simulink model "boost_simulink_copy"  (R2021a)
settings: Solver=FixedStepDiscrete  StartTime=0.0  StopTime=0.5  FixedStep=sampleTime  MaxStep=1e-4  RelTol=1e-4  EnableMultiTasking=on
InitFcn:
  | boost_parameters
model workspace (MAT data in the model file):
  Phase1 = 0
values from neighbouring files (symbols this model uses):
  CoutModulesp = 271e-6    (= 0.000271)    [boost_parameters.m]    (also in unbalance_boost.m)
  D = (1-Vin/Vout)    (= 0.25)    [boost_parameters.m]    (also in calculations.m = (1-VinOneModule/VoutOneModule); flying_capacitor_parameters.m; unbalance_boost.m)
  Lcoilsp = 0.517e-3    (= 0.000517)    [boost_parameters.m]    (also in unbalance_boost.m = 0.001034)
  ModuleAPhase = 0    [boost_parameters.m]    (also in flying_capacitor_parameters.m = 90; unbalance_boost.m)
  ModuleBPhase = 180    [boost_parameters.m]    (also in flying_capacitor_parameters.m = 270; unbalance_boost.m = 90)
  ModuleCPhase = 180    [boost_parameters.m]    (also in flying_capacitor_parameters.m = 0)
  ModuleDPhase = 180    [boost_parameters.m]    (also in flying_capacitor_parameters.m)
  Rcoil = 1e-3    (= 0.001)    [boost_parameters.m]    (also in unbalance_boost.m)
  sampleTime = 5e-8    (= 5e-08)    [boost_parameters.m]    (also in flying_capacitor_parameters.m = 5e-07; unbalance_boost.m)
  Vin = 900    [boost_parameters.m]    (also in flying_capacitor_parameters.m; main.m = 880; unbalance_boost.m)
libraries: spsSeriesRLCBranchLib x35, spsVoltageMeasurementLib x32, spsCurrentMeasurementLib x27, spsDiodeLib x14, spsIGBTDiodeLib x14, simulink x10, spsDCVoltageSourceLib x7, spsTriangleGeneratorLib x5, spspowerguiLib x2
settings Model: Creator=The MathWorks, Inc.  LastModifiedBy=enes_
settings SolverCC: AlgebraicLoopSolver=TrustRegion  SolverResetMethod=Robust
settings OptimizationCC: EfficientFloat2IntCast=on  LifeSpan=inf
settings DebuggingCC: ReadBeforeWriteMsg=DisableAll  WriteAfterWriteMsg=DisableAll  WriteAfterReadMsg=DisableAll  UniqueDataStoreMsg=error  StrictBusMsg=ErrorOnBusTreatedAsVector  SFUnexpectedBacktrackingDiag=warning  SFNoUnconditionalDefaultTransitionDiag=warning  SFExecutionAtInitializationDiag=none  SFMachineParentedDataDiag=warning  ArithmeticOperatorsInVariantConditions=warning
settings ModelReferenceCC: UpdateModelReferenceTargets=IfOutOfDate
settings SFSimCC: SFSimEcho=off  SimUseLocalCustomCode=off  CustomCodeUndefinedFunction=UseInterfaceOnly
settings RTWCC: RTWUseLocalCustomCode=off
settings CodeAppCC: StateflowObjectComments=on
settings GRTTargetCC: TargetLangStandard=C89/C90 (ANSI)
settings ConfigComp: CovMetricSettings=dw  CovSaveCumulativeToWorkspaceVar=on  CovSaveSingleToWorkspaceVar=on  CovExternalEMLEnable=off
settings SimscapeCC: SimscapeNormalizeSystem=off  SimscapeNominalValues={1, 'bar'; 1, 'cm^3/s'; 1, 'bar*kg/s'; 1, 'kJ/kg'; 1, 'kW'; }

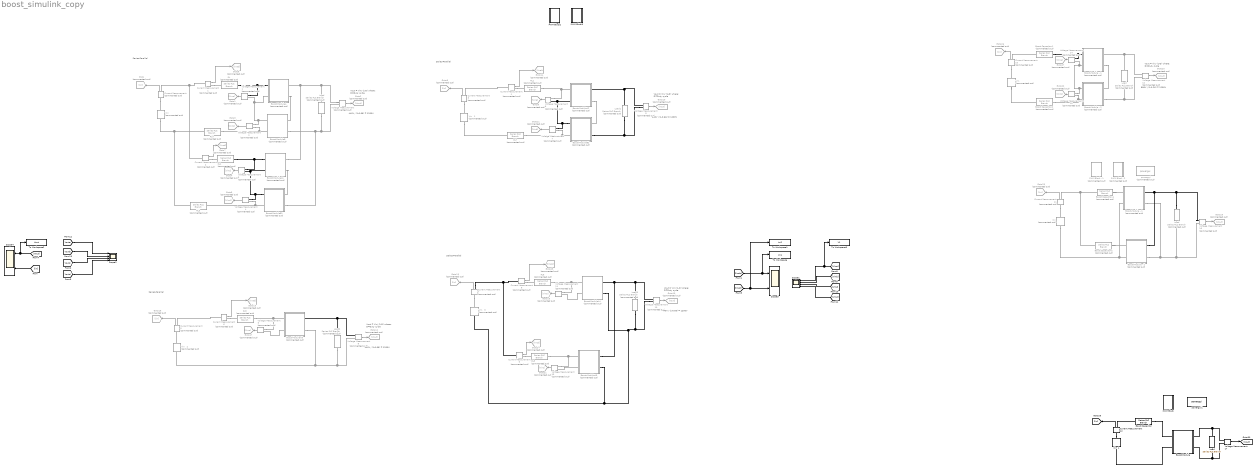
== system boost_simulink_copy ==
  note: Series-Parallel
  note: Vout = Vin/ (1-D)
      | where: D=Duty cycle
  note: 440V / (1-0.66) = 1200V
  note: Series-Parallel
  note: Vout = Vin/ (1-D)
      | where: D=Duty cycle
  note: 440V / (1-0.66) = 1200V
  note: 440V / (1-0.66) = 1200V
  note: Vout = Vin/ (1-D)
      | where: D=Duty cycle
  note: Series-Parallel
  note: Series-Parallel
  note: Vout = Vin/ (1-D)
      | where: D=Duty cycle
  note: 440V / (1-0.66) = 1200V
  note: 880V / (1-0.26) = 1200V
  note: Vout = Vin/ (1-D)
      | where: D=Duty cycle
  "Boost Capacitor   " : spsSeriesRLCBranchLib/Series RLC Branch  LConnTagsString=__new0  RConnTagsString=__new0  BranchType=L  Resistance=Rcoil  Inductance=Lcoilsp*2  SetiL0=off  InitialCurrent=8  Capacitance=1e-6  Setx0=off  InitialVoltage=0  Measurements=None
  Boost Capacitor-1 : spsSeriesRLCBranchLib/Series RLC Branch  Commented=on  LConnTagsString=__new0  RConnTagsString=__new0  BranchType=L  Resistance=Rcoil  Inductance=Lcoilsp/2  SetiL0=off  InitialCurrent=8  Capacitance=1e-6  Setx0=off  InitialVoltage=0  Measurements=None
  "Boost Capacitor-1  " : spsSeriesRLCBranchLib/Series RLC Branch  Commented=on  LConnTagsString=__new0  RConnTagsString=__new0  BranchType=L  Resistance=Rcoil  Inductance=Lcoilsp*2  SetiL0=off  InitialCurrent=8  Capacitance=1e-6  Setx0=off  InitialVoltage=0  Measurements=None
  Boost Capacitor-2 : spsSeriesRLCBranchLib/Series RLC Branch  Commented=on  LConnTagsString=__new0  RConnTagsString=__new0  BranchType=L  Resistance=Rcoil  Inductance=Lcoilsp/2  SetiL0=off  InitialCurrent=8  Capacitance=1e-6  Setx0=off  InitialVoltage=0  Measurements=None
  "Boost Capacitor-2   " : spsSeriesRLCBranchLib/Series RLC Branch  Commented=on  LConnTagsString=__new0  RConnTagsString=__new0  BranchType=L  Resistance=Rcoil  Inductance=Lcoilsp*2  SetiL0=off  InitialCurrent=8  Capacitance=1e-6  Setx0=off  InitialVoltage=0  Measurements=None
  "Boost-Module      " : Subsystem
  Boost-Module - 1 : Subsystem  Commented=on
  "Boost-Module - 1  " : Subsystem  Commented=on
  Boost-Module - 2 : Subsystem  Commented=on
  "Boost-Module - 2  " : Subsystem  Commented=on
  Boost-ModuleA : Subsystem  Commented=on
  Boost-ModuleA1 : Subsystem  Commented=on
  Boost-ModuleA2 : Subsystem  Commented=on
  Boost-ModuleA3 : Subsystem  Commented=on
  Boost-ModuleA4 : Subsystem  Commented=on
  Boost-ModuleA5 : Subsystem  Commented=on
  Boost-ModuleB : Subsystem  Commented=on
  Boost-ModuleB1 : Subsystem  Commented=on
  Boost-ModuleB2 : Subsystem  Commented=on
  Current Measurement{,1..11} (12 alike) : spsCurrentMeasurementLib/Current Measurement  Commented=on  PhasorSimulation=off  OutputType=Complex  PSBequivalent=0
  Current Measurement12 : spsCurrentMeasurementLib/Current Measurement  PhasorSimulation=off  OutputType=Complex  PSBequivalent=0
  Goto{,8,13,16,25..26} (6 alike) : Goto  Commented=on  GotoTag=Iin
  Goto{1,9,17..18,27} (5 alike) : Goto  Commented=on  GotoTag=Vina
  Goto{2,10,12,19..20,29} (6 alike) : Goto  Commented=on  GotoTag=Vout
  Goto11 : Goto  Commented=on  GotoTag=Vinb
  Goto{6,14..15,23} (4 alike) : Goto  Commented=on  GotoTag=Iinab
  Goto21 : Goto  Commented=on  GotoTag=Vinc
  Goto22 : Goto  Commented=on  GotoTag=Vinb
  Goto24 : Goto  Commented=on  GotoTag=Iincd
  Goto3 : Goto  Commented=on  GotoTag=Vinb
  Goto4 : Goto  Commented=on  GotoTag=Vinc
  Goto5 : Goto  Commented=on  GotoTag=Vind
  Goto7 : Goto  Commented=on  GotoTag=Iincd
  Load{,1..3} (4 alike) : spsSeriesRLCBranchLib/Series RLC Branch  Commented=on  LConnTagsString=__new0  RConnTagsString=__new0  BranchType=R  Resistance=72  Inductance=200e-6  SetiL0=off  InitialCurrent=0  Capacitance=400e-6  Setx0=off  InitialVoltage=0  Measurements=None
  "Load  " : spsSeriesRLCBranchLib/Series RLC Branch  Commented=on  LConnTagsString=__new0  RConnTagsString=__new0  BranchType=R  Resistance=72  Inductance=200e-6  SetiL0=off  InitialCurrent=0  Capacitance=400e-6  Setx0=off  InitialVoltage=0  Measurements=None
  "Load    " : spsSeriesRLCBranchLib/Series RLC Branch  Commented=on  LConnTagsString=__new0  RConnTagsString=__new0  BranchType=R  Resistance=72  Inductance=200e-6  SetiL0=off  InitialCurrent=0  Capacitance=400e-6  Setx0=off  InitialVoltage=0  Measurements=None
  "Load     " : spsSeriesRLCBranchLib/Series RLC Branch  LConnTagsString=__new0  RConnTagsString=__new0  BranchType=R  Resistance=72  Inductance=200e-6  SetiL0=off  InitialCurrent=0  Capacitance=400e-6  Setx0=off  InitialVoltage=0  Measurements=None
  "PWM Block " : Subsystem
  PWM Block - 1 : Subsystem  Commented=on
  PWM Block - 2 : Subsystem  Commented=on
  PWM Block2 : Subsystem
  PWM Block3 : Subsystem
  RL{,1,3..4} (4 alike) : spsSeriesRLCBranchLib/Series RLC Branch  Commented=on  LConnTagsString=__new0  RConnTagsString=__new0  BranchType=L  Resistance=Rcoil  Inductance=Lcoilsp  SetiL0=off  InitialCurrent=8  Capacitance=1e-6  Setx0=off  InitialVoltage=0  Measurements=None
  RL2 : spsSeriesRLCBranchLib/Series RLC Branch  Commented=on  LConnTagsString=__new0  RConnTagsString=__new0  BranchType=L  Resistance=Rcoil  Inductance=Lcoilsp/2  SetiL0=off  InitialCurrent=8  Capacitance=1e-6  Setx0=off  InitialVoltage=0  Measurements=None
  RL5 : spsSeriesRLCBranchLib/Series RLC Branch  Commented=on  LConnTagsString=__new0  RConnTagsString=__new0  BranchType=L  Resistance=Rcoil  Inductance=Lcoilsp*2  SetiL0=off  InitialCurrent=8  Capacitance=1e-6  Setx0=off  InitialVoltage=0  Measurements=None
  RL6 : spsSeriesRLCBranchLib/Series RLC Branch  Commented=on  LConnTagsString=__new0  RConnTagsString=__new0  BranchType=L  Resistance=Rcoil  Inductance=Lcoilsp*2  SetiL0=off  InitialCurrent=8  Capacitance=1e-6  Setx0=off  InitialVoltage=0  Measurements=None
  RL7 : spsSeriesRLCBranchLib/Series RLC Branch  Commented=on  LConnTagsString=__new0  RConnTagsString=__new0  BranchType=L  Resistance=Rcoil  Inductance=Lcoilsp/2  SetiL0=off  InitialCurrent=8  Capacitance=1e-6  Setx0=off  InitialVoltage=0  Measurements=None
  RL8 : spsSeriesRLCBranchLib/Series RLC Branch  Commented=on  LConnTagsString=__new0  RConnTagsString=__new0  BranchType=L  Resistance=Rcoil  Inductance=Lcoilsp*2  SetiL0=off  InitialCurrent=8  Capacitance=1e-6  Setx0=off  InitialVoltage=0  Measurements=None
  Scope1 : Scope  NumInputPorts=4
  Scope2 : Scope  NumInputPorts=4
  Scope3 : Scope  NumInputPorts=2
  Scope4 : Scope  NumInputPorts=2
  To Workspace : ToWorkspace  VariableName=Im1  SaveFormat=Timeseries  SampleTime=-1
  To Workspace1 : ToWorkspace  VariableName=Im2  SaveFormat=Timeseries  SampleTime=-1
  To Workspace2 : ToWorkspace  VariableName=Vout  SaveFormat=Timeseries  SampleTime=-1
  To Workspace3 : ToWorkspace  VariableName=V1  SaveFormat=Timeseries  SampleTime=-1
  "Vin  " : spsDCVoltageSourceLib/DC Voltage Source  Commented=on  Amplitude=Vin  Measurements=None
  Vin   {,1..3} (4 alike) : spsDCVoltageSourceLib/DC Voltage Source  Commented=on  Amplitude=Vin  Measurements=None
  "Vin     " : spsDCVoltageSourceLib/DC Voltage Source  Commented=on  Amplitude=Vin  Measurements=None
  Vin  1 : spsDCVoltageSourceLib/DC Voltage Source  Amplitude=Vin  Measurements=None
  Voltage Measurement{,1..16} (17 alike) : spsVoltageMeasurementLib/Voltage Measurement  Commented=on  PhasorSimulation=off  OutputType=Complex  PSBequivalent=0
  Voltage Measurement17 : spsVoltageMeasurementLib/Voltage Measurement  PhasorSimulation=off  OutputType=Complex  PSBequivalent=0
  powergui : spspowerguiLib/powergui  Priority=1  Commented=on  SimulationMode=Discrete  SampleTime=sampleTime  frequency=60  Iterations=50  frequencyindice=0  Pbase=100e6  ErrMax=1e-4  UnitsV=kV  UnitsW=MW  buscounter=0  FunctionMessages=off  echomessages=off  EnableUseOfTLC=off  CurrentSourceSwitches=off  DisableSnubberDevices=off  DisableRonSwitches=off  DisableVfSwitches=off  DisplayEquations=off  AutomaticDiscreteSolvers=off  SolverType=Tustin/Backward Euler (TBE)  Interpol=off  ExternalGateDelay=off  methode=off  Ts=100  x0status=blocks  SPID=on  SwTol=0  HookPort=off  NonlinearTolerance=1e-4  nMaxIteration=100  ContinueOnMaxIteration=off  RestoreLinks=warning  ResistiveCurrentMeasurement=off  Frange=[0:2:500]  Ylog=off  Xlog=on  ShowGrid=off  save=off  variable=ZData  structure=0  ZoomFFT=off  StartTime=0.0  cycles=1  DisplayStyle=1  fundamental=60  FreqAxis=off  MaxFrequency=1000  frequencyindicesteady=1  RmsSteady=1  display=off
  powergui1 : spspowerguiLib/powergui  Priority=1  SimulationMode=Discrete  SampleTime=sampleTime  frequency=60  Iterations=50  frequencyindice=0  Pbase=100e6  ErrMax=1e-4  UnitsV=kV  UnitsW=MW  buscounter=0  FunctionMessages=off  echomessages=off  EnableUseOfTLC=off  CurrentSourceSwitches=off  DisableSnubberDevices=off  DisableRonSwitches=off  DisableVfSwitches=off  DisplayEquations=off  AutomaticDiscreteSolvers=off  SolverType=Tustin/Backward Euler (TBE)  Interpol=off  ExternalGateDelay=off  methode=off  Ts=100  x0status=blocks  SPID=on  SwTol=0  HookPort=off  NonlinearTolerance=1e-4  nMaxIteration=100  ContinueOnMaxIteration=off  RestoreLinks=warning  ResistiveCurrentMeasurement=off  Frange=[0:2:500]  Ylog=off  Xlog=on  ShowGrid=off  save=off  variable=ZData  structure=0  ZoomFFT=off  StartTime=0.0  cycles=1  DisplayStyle=1  fundamental=60  FreqAxis=off  MaxFrequency=1000  frequencyindicesteady=1  RmsSteady=1  display=off
  wires:
  [Vout] -> To Workspace2/1, Scope4/1  "Vout"
  [Iin] -> Scope4/2
  [Vina] -> To Workspace3/1, Scope1/1
  [Vinb] -> Scope1/2
  [Vinc] -> Scope1/3
  [Vind] -> Scope1/4
  [Iincd] -> To Workspace1/1, Scope3/2
  [Iinab] -> Scope3/1, To Workspace/1
  [Vouta] -> Scope2/1  "A"
  [Voutb] -> Scope2/2  "B"
  [Voutc] -> Scope2/3  "C"
  [Voutd] -> Scope2/4  "D"
  Current Measurement2/1 -> Goto7/1
  Current Measurement1/1 -> Goto6/1
  Voltage Measurement2/1 -> Goto3/1
  Voltage Measurement4/1 -> Goto5/1
  Voltage Measurement3/1 -> Goto4/1
  Voltage Measurement1/1 -> Goto1/1
  Current Measurement/1 -> Goto/1
  Voltage Measurement/1 -> Goto2/1
  Voltage Measurement7/1 -> Goto11/1
  Voltage Measurement5/1 -> Goto10/1
  Voltage Measurement6/1 -> Goto9/1
  Current Measurement3/1 -> Goto8/1
  Current Measurement4/1 -> Goto14/1
  Voltage Measurement8/1 -> Goto12/1
  Current Measurement6/1 -> Goto15/1
  Current Measurement5/1 -> Goto16/1
  Voltage Measurement9/1 -> Goto17/1
  Current Measurement9/1 -> Goto24/1
  Voltage Measurement10/1 -> Goto19/1
  Voltage Measurement11/1 -> Goto18/1
  Current Measurement7/1 -> Goto13/1
  Current Measurement8/1 -> Goto23/1
  Voltage Measurement13/1 -> Goto21/1
  Voltage Measurement15/1 -> Goto22/1
  Voltage Measurement14/1 -> Goto27/1
  Current Measurement10/1 -> Goto26/1
  Voltage Measurement12/1 -> Goto20/1
  Current Measurement11/1 -> Goto25/1
  Voltage Measurement16/1 -> Goto29/1
  Voltage Measurement17/1 -> [Vout]
  Current Measurement12/1 -> [Iin]
  connections:
  Current Measurement2/RConn1 -- RL1/LConn1
  Boost-ModuleA/RConn2 -- Boost-ModuleB/RConn1
  Current Measurement1/RConn1 -- RL/LConn1
  Boost-ModuleA1/RConn2 -- Boost-ModuleB1/RConn1
  Boost-ModuleA/LConn1 -- RL/RConn1 -- Voltage Measurement1/LConn1
  Boost-ModuleA1/LConn1 -- RL1/RConn1 -- Voltage Measurement3/LConn1
  Current Measurement1/LConn1 -- Current Measurement2/LConn1 -- Current Measurement/RConn1
  Boost-ModuleB/RConn2 -- Boost-ModuleB1/RConn2 -- Load/RConn1 -- Voltage Measurement/LConn2
  Boost-ModuleA/LConn2 -- Voltage Measurement2/LConn1 -- Boost-ModuleB/LConn1 -- Voltage Measurement1/LConn2
  Boost-ModuleB1/LConn1 -- Boost-ModuleA1/LConn2 -- Voltage Measurement3/LConn2 -- Voltage Measurement4/LConn1
  Voltage Measurement2/LConn2 -- RL4/RConn1 -- Boost-ModuleB/LConn2
  Voltage Measurement/LConn1 -- Load/LConn1 -- Boost-ModuleA1/RConn1 -- Boost-ModuleA/RConn1
  Current Measurement/LConn1 -- "Vin   "/RConn1
  Boost-ModuleB1/LConn2 -- Voltage Measurement4/LConn2 -- RL3/RConn1
  RL3/LConn1 -- "Vin   "/LConn1 -- RL4/LConn1
  Boost-ModuleA2/RConn1 -- Voltage Measurement5/LConn1 -- Load1/LConn1
  Voltage Measurement6/LConn1 -- RL2/RConn1 -- Boost-ModuleA2/LConn1
  Voltage Measurement5/LConn2 -- Boost-ModuleB2/RConn2 -- Load1/RConn1
  Boost-ModuleB2/LConn1 -- Boost-ModuleA2/LConn2 -- Voltage Measurement6/LConn2 -- Voltage Measurement7/LConn1
  Boost-ModuleB2/LConn2 -- Voltage Measurement7/LConn2 -- RL7/RConn1
  Current Measurement4/LConn1 -- Current Measurement3/RConn1
  Vin   1/LConn1 -- RL7/LConn1
  Current Measurement4/RConn1 -- RL2/LConn1
  Boost-ModuleA2/RConn2 -- Boost-ModuleB2/RConn1
  Current Measurement3/LConn1 -- Vin   1/RConn1
  Boost-ModuleA3/LConn2 -- Voltage Measurement9/LConn2
  Boost-ModuleA3/RConn1 -- Voltage Measurement8/LConn1 -- Load2/LConn1
  Voltage Measurement9/LConn1 -- Boost-ModuleA3/LConn1 -- RL5/RConn1
  Current Measurement6/RConn1 -- RL5/LConn1
  Load2/RConn1 -- Vin   2/LConn1 -- Boost-ModuleA3/RConn2 -- Voltage Measurement8/LConn2
  Current Measurement6/LConn1 -- Current Measurement5/RConn1
  Boost-ModuleA4/RConn1 -- Boost-ModuleA5/RConn1 -- Voltage Measurement10/LConn1 -- Load3/LConn1
  Voltage Measurement11/LConn1 -- Boost-ModuleA4/LConn1 -- RL6/RConn1
  Voltage Measurement10/LConn2 -- Boost-ModuleA4/RConn2 -- Vin   3/LConn1 -- Boost-ModuleA5/RConn2 -- Load3/RConn1
  Boost-ModuleA4/LConn2 -- Voltage Measurement11/LConn2
  Boost-ModuleA5/LConn2 -- Voltage Measurement13/LConn2
  Current Measurement7/RConn1 -- Current Measurement8/LConn1 -- Current Measurement9/LConn1
  Voltage Measurement13/LConn1 -- Boost-ModuleA5/LConn1 -- RL8/RConn1
  Current Measurement8/RConn1 -- RL6/LConn1
  Current Measurement7/LConn1 -- Vin   3/RConn1
  Current Measurement9/RConn1 -- RL8/LConn1
  Vin   2/RConn1 -- Current Measurement5/LConn1
  Boost Capacitor-2/RConn1 -- Boost-Module - 2/LConn2 -- Voltage Measurement15/LConn2
  "Load  "/RConn1 -- Voltage Measurement12/LConn2 -- Boost-Module - 2/RConn2
  Voltage Measurement15/LConn1 -- Boost-Module - 1/LConn2 -- Voltage Measurement14/LConn2 -- Boost-Module - 2/LConn1
  Voltage Measurement12/LConn1 -- "Load  "/LConn1 -- Boost-Module - 1/RConn1
  Boost-Module - 1/LConn1 -- Boost Capacitor-1/RConn1 -- Voltage Measurement14/LConn1
  Current Measurement10/RConn1 -- Boost Capacitor-1/LConn1
  Current Measurement10/LConn1 -- "Vin     "/RConn1
  "Vin     "/LConn1 -- Boost Capacitor-2/LConn1
  Boost-Module - 1/RConn2 -- Boost-Module - 2/RConn1
  "Load    "/RConn1 -- "Boost-Module - 1  "/RConn2 -- "Boost-Module - 2  "/RConn2 -- Voltage Measurement16/LConn2
  "Boost Capacitor-2   "/RConn1 -- "Boost-Module - 2  "/LConn1
  "Boost Capacitor-1  "/RConn1 -- "Boost-Module - 1  "/LConn1
  "Load    "/LConn1 -- Voltage Measurement16/LConn1 -- "Boost-Module - 1  "/RConn1 -- "Boost-Module - 2  "/RConn1
  Current Measurement11/LConn1 -- "Vin  "/RConn1
  "Boost-Module - 1  "/LConn2 -- "Vin  "/LConn1 -- "Boost-Module - 2  "/LConn2
  Current Measurement11/RConn1 -- "Boost Capacitor-2   "/LConn1 -- "Boost Capacitor-1  "/LConn1
  Current Measurement12/RConn1 -- "Boost Capacitor   "/LConn1
  Voltage Measurement17/LConn1 -- "Load     "/LConn1 -- "Boost-Module      "/RConn1
  "Load     "/RConn1 -- "Boost-Module      "/RConn2 -- Voltage Measurement17/LConn2
  "Boost Capacitor   "/RConn1 -- "Boost-Module      "/LConn1
  Current Measurement12/LConn1 -- Vin  1/RConn1
  Vin  1/LConn1 -- "Boost-Module      "/LConn2

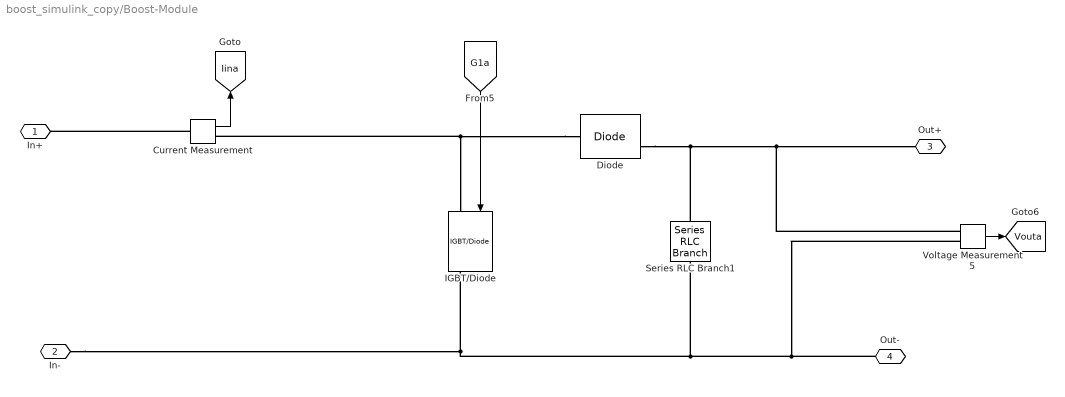
== system boost_simulink_copy/Boost-Module       ==
  Current Measurement : spsCurrentMeasurementLib/Current Measurement  PhasorSimulation=off  OutputType=Complex  PSBequivalent=0
  Diode : spsDiodeLib/Diode  Ron=0.001  Lon=0  Vf=0.8  IC=0  UseSnubber=0  Rs=500  Cs=250e-9  Measurements=on
  IGBT/Diode : spsIGBTDiodeLib/IGBT//Diode  Ron=1e-3  Rs=1e5  Cs=inf  Measurements=on
  Series RLC Branch1 : spsSeriesRLCBranchLib/Series RLC Branch  LConnTagsString=__new0  RConnTagsString=__new0  BranchType=C  Resistance=1e-4  Inductance=200e-6  SetiL0=off  InitialCurrent=0  Capacitance=CoutModulesp  Setx0=off  InitialVoltage=1200  Measurements=None
  Voltage Measurement5 : spsVoltageMeasurementLib/Voltage Measurement  PhasorSimulation=off  OutputType=Complex  PSBequivalent=0
  In+ : PMIOPort  Side=Left
  In- : PMIOPort  Port=2  Side=Left
  Out+ : PMIOPort  Port=3  Side=Right
  Out- : PMIOPort  Port=4  Side=Right
  tag scope: Iina=global, Vouta=global
  wires:
  [G1a] -> IGBT/Diode/1
  Current Measurement/1 -> [Iina]
  Voltage Measurement5/1 -> [Vouta]
  connections:
  Diode/LConn1 -- IGBT/Diode/LConn1 -- Current Measurement/RConn1
  Series RLC Branch1/LConn1 -- Diode/RConn1 -- Voltage Measurement5/LConn1 -- Out+/RConn1
  Current Measurement/LConn1 -- In+/RConn1
  Out-/RConn1 -- Voltage Measurement5/LConn2 -- In-/RConn1 -- IGBT/Diode/RConn1 -- Series RLC Branch1/RConn1

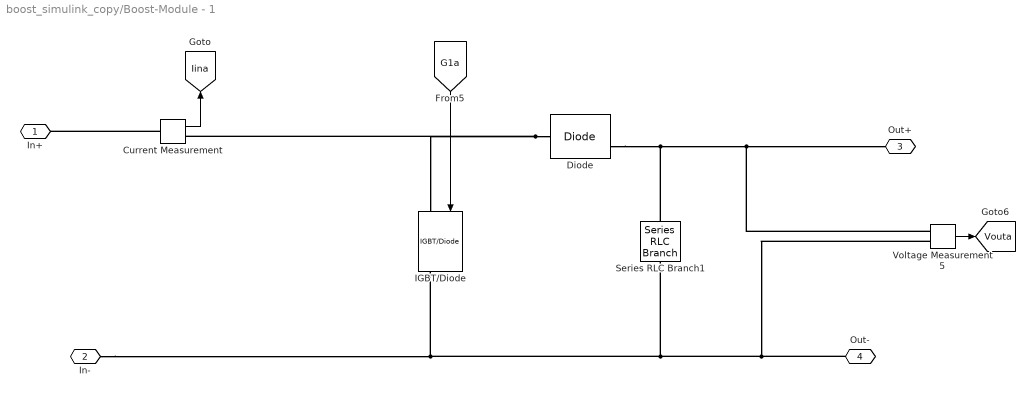
== system boost_simulink_copy/Boost-Module - 1 ==
  Current Measurement : spsCurrentMeasurementLib/Current Measurement  PhasorSimulation=off  OutputType=Complex  PSBequivalent=0
  Diode : spsDiodeLib/Diode  Ron=0.001  Lon=0  Vf=0.8  IC=0  UseSnubber=0  Rs=500  Cs=250e-9  Measurements=on
  IGBT/Diode : spsIGBTDiodeLib/IGBT//Diode  Ron=1e-3  Rs=1e5  Cs=inf  Measurements=on
  Series RLC Branch1 : spsSeriesRLCBranchLib/Series RLC Branch  LConnTagsString=__new0  RConnTagsString=__new0  BranchType=C  Resistance=1e-4  Inductance=200e-6  SetiL0=off  InitialCurrent=0  Capacitance=CoutModulesp  Setx0=off  InitialVoltage=1200  Measurements=None
  Voltage Measurement5 : spsVoltageMeasurementLib/Voltage Measurement  PhasorSimulation=off  OutputType=Complex  PSBequivalent=0
  In+ : PMIOPort  Side=Left
  In- : PMIOPort  Port=2  Side=Left
  Out+ : PMIOPort  Port=3  Side=Right
  Out- : PMIOPort  Port=4  Side=Right
  tag scope: Iina=global, Vouta=global
  wires:
  [G1a] -> IGBT/Diode/1
  Current Measurement/1 -> [Iina]
  Voltage Measurement5/1 -> [Vouta]
  connections:
  Diode/LConn1 -- IGBT/Diode/LConn1 -- Current Measurement/RConn1
  Series RLC Branch1/LConn1 -- Diode/RConn1 -- Voltage Measurement5/LConn1 -- Out+/RConn1
  Current Measurement/LConn1 -- In+/RConn1
  Out-/RConn1 -- Voltage Measurement5/LConn2 -- IGBT/Diode/RConn1 -- In-/RConn1 -- Series RLC Branch1/RConn1

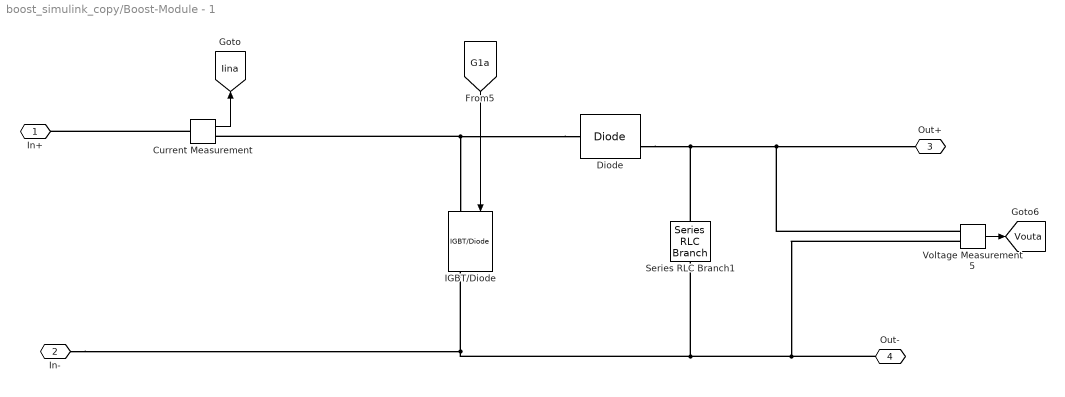
== system boost_simulink_copy/Boost-Module - 1   ==
  Current Measurement : spsCurrentMeasurementLib/Current Measurement  PhasorSimulation=off  OutputType=Complex  PSBequivalent=0
  Diode : spsDiodeLib/Diode  Ron=0.001  Lon=0  Vf=0.8  IC=0  UseSnubber=0  Rs=500  Cs=250e-9  Measurements=on
  IGBT/Diode : spsIGBTDiodeLib/IGBT//Diode  Ron=1e-3  Rs=1e5  Cs=inf  Measurements=on
  Series RLC Branch1 : spsSeriesRLCBranchLib/Series RLC Branch  LConnTagsString=__new0  RConnTagsString=__new0  BranchType=C  Resistance=1e-4  Inductance=200e-6  SetiL0=off  InitialCurrent=0  Capacitance=CoutModulesp  Setx0=off  InitialVoltage=1200  Measurements=None
  Voltage Measurement5 : spsVoltageMeasurementLib/Voltage Measurement  PhasorSimulation=off  OutputType=Complex  PSBequivalent=0
  In+ : PMIOPort  Side=Left
  In- : PMIOPort  Port=2  Side=Left
  Out+ : PMIOPort  Port=3  Side=Right
  Out- : PMIOPort  Port=4  Side=Right
  tag scope: Iina=global, Vouta=global
  wires:
  [G1a] -> IGBT/Diode/1
  Current Measurement/1 -> [Iina]
  Voltage Measurement5/1 -> [Vouta]
  connections:
  Diode/LConn1 -- IGBT/Diode/LConn1 -- Current Measurement/RConn1
  Series RLC Branch1/LConn1 -- Diode/RConn1 -- Voltage Measurement5/LConn1 -- Out+/RConn1
  Current Measurement/LConn1 -- In+/RConn1
  Out-/RConn1 -- Voltage Measurement5/LConn2 -- In-/RConn1 -- IGBT/Diode/RConn1 -- Series RLC Branch1/RConn1

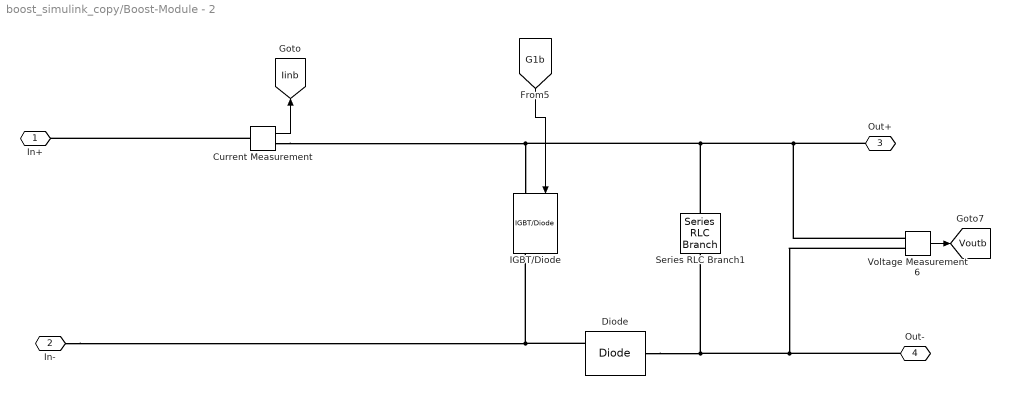
== system boost_simulink_copy/Boost-Module - 2 ==
  Current Measurement : spsCurrentMeasurementLib/Current Measurement  PhasorSimulation=off  OutputType=Complex  PSBequivalent=0
  Diode : spsDiodeLib/Diode  Ron=0.001  Lon=0  Vf=0.8  IC=0  UseSnubber=0  Rs=500  Cs=250e-9  Measurements=on
  IGBT/Diode : spsIGBTDiodeLib/IGBT//Diode  Ron=1e-3  Rs=1e5  Cs=inf  Measurements=on
  Series RLC Branch1 : spsSeriesRLCBranchLib/Series RLC Branch  LConnTagsString=__new0  RConnTagsString=__new0  BranchType=C  Resistance=1e-4  Inductance=200e-6  SetiL0=off  InitialCurrent=0  Capacitance=CoutModulesp  Setx0=off  InitialVoltage=1200  Measurements=None
  Voltage Measurement6 : spsVoltageMeasurementLib/Voltage Measurement  PhasorSimulation=off  OutputType=Complex  PSBequivalent=0
  In+ : PMIOPort  Side=Left
  In- : PMIOPort  Port=2  Side=Left
  Out+ : PMIOPort  Port=3  Side=Right
  Out- : PMIOPort  Port=4  Side=Right
  tag scope: Iinb=global, Voutb=global
  wires:
  Current Measurement/1 -> [Iinb]
  [G1b] -> IGBT/Diode/1
  Voltage Measurement6/1 -> [Voutb]
  connections:
  Out+/RConn1 -- Voltage Measurement6/LConn1 -- Series RLC Branch1/LConn1 -- Current Measurement/RConn1 -- IGBT/Diode/LConn1
  Out-/RConn1 -- Voltage Measurement6/LConn2 -- Diode/LConn1 -- Series RLC Branch1/RConn1
  Current Measurement/LConn1 -- In+/RConn1
  In-/RConn1 -- Diode/RConn1 -- IGBT/Diode/RConn1

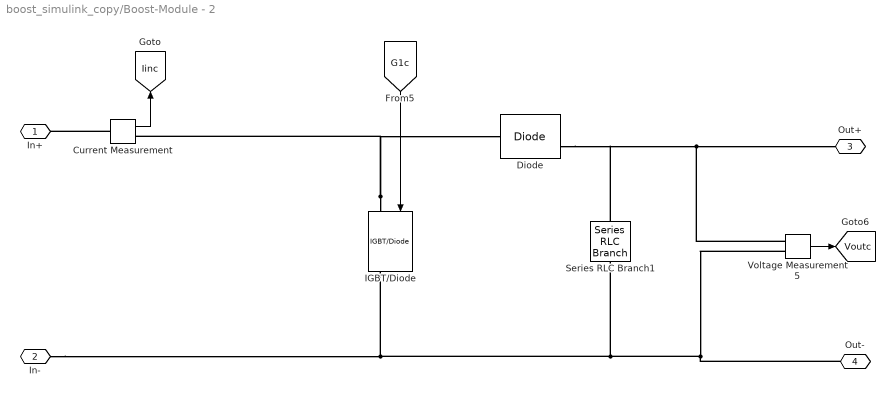
== system boost_simulink_copy/Boost-Module - 2   ==
  Current Measurement : spsCurrentMeasurementLib/Current Measurement  PhasorSimulation=off  OutputType=Complex  PSBequivalent=0
  Diode : spsDiodeLib/Diode  Ron=0.001  Lon=0  Vf=0.8  IC=0  UseSnubber=0  Rs=500  Cs=250e-9  Measurements=on
  IGBT/Diode : spsIGBTDiodeLib/IGBT//Diode  Ron=1e-3  Rs=1e5  Cs=inf  Measurements=on
  Series RLC Branch1 : spsSeriesRLCBranchLib/Series RLC Branch  LConnTagsString=__new0  RConnTagsString=__new0  BranchType=C  Resistance=1e-4  Inductance=200e-6  SetiL0=off  InitialCurrent=0  Capacitance=CoutModulesp  Setx0=off  InitialVoltage=1200  Measurements=None
  Voltage Measurement5 : spsVoltageMeasurementLib/Voltage Measurement  PhasorSimulation=off  OutputType=Complex  PSBequivalent=0
  In+ : PMIOPort  Side=Left
  In- : PMIOPort  Port=2  Side=Left
  Out+ : PMIOPort  Port=3  Side=Right
  Out- : PMIOPort  Port=4  Side=Right
  tag scope: Iinc=global, Voutc=global
  wires:
  [G1c] -> IGBT/Diode/1
  Current Measurement/1 -> [Iinc]
  Voltage Measurement5/1 -> [Voutc]
  connections:
  IGBT/Diode/LConn1 -- Diode/LConn1 -- Current Measurement/RConn1
  Voltage Measurement5/LConn1 -- Out+/RConn1 -- Series RLC Branch1/LConn1 -- Diode/RConn1
  Current Measurement/LConn1 -- In+/RConn1
  Voltage Measurement5/LConn2 -- Out-/RConn1 -- Series RLC Branch1/RConn1 -- In-/RConn1 -- IGBT/Diode/RConn1

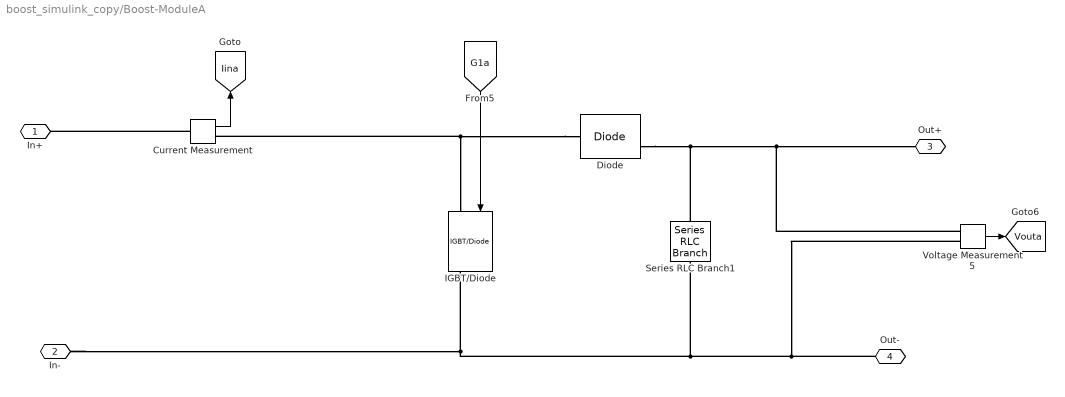
== system boost_simulink_copy/Boost-ModuleA ==
  Current Measurement : spsCurrentMeasurementLib/Current Measurement  PhasorSimulation=off  OutputType=Complex  PSBequivalent=0
  Diode : spsDiodeLib/Diode  Ron=0.001  Lon=0  Vf=0.8  IC=0  UseSnubber=0  Rs=500  Cs=250e-9  Measurements=on
  IGBT/Diode : spsIGBTDiodeLib/IGBT//Diode  Ron=1e-3  Rs=1e5  Cs=inf  Measurements=on
  Series RLC Branch1 : spsSeriesRLCBranchLib/Series RLC Branch  LConnTagsString=__new0  RConnTagsString=__new0  BranchType=C  Resistance=1e-4  Inductance=200e-6  SetiL0=off  InitialCurrent=0  Capacitance=CoutModulesp  Setx0=off  InitialVoltage=1200  Measurements=None
  Voltage Measurement5 : spsVoltageMeasurementLib/Voltage Measurement  PhasorSimulation=off  OutputType=Complex  PSBequivalent=0
  In+ : PMIOPort  Side=Left
  In- : PMIOPort  Port=2  Side=Left
  Out+ : PMIOPort  Port=3  Side=Right
  Out- : PMIOPort  Port=4  Side=Right
  tag scope: Iina=global, Vouta=global
  wires:
  [G1a] -> IGBT/Diode/1
  Current Measurement/1 -> [Iina]
  Voltage Measurement5/1 -> [Vouta]
  connections:
  Diode/LConn1 -- IGBT/Diode/LConn1 -- Current Measurement/RConn1
  Series RLC Branch1/LConn1 -- Diode/RConn1 -- Voltage Measurement5/LConn1 -- Out+/RConn1
  Current Measurement/LConn1 -- In+/RConn1
  Out-/RConn1 -- Voltage Measurement5/LConn2 -- In-/RConn1 -- IGBT/Diode/RConn1 -- Series RLC Branch1/RConn1

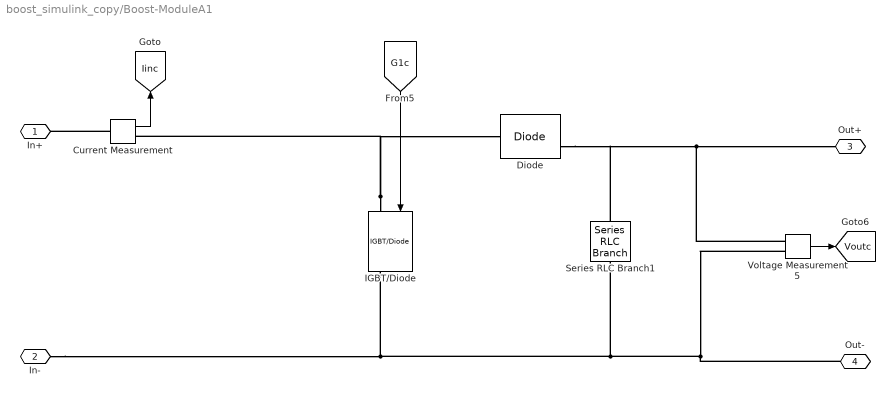
== system boost_simulink_copy/Boost-ModuleA1 ==
  Current Measurement : spsCurrentMeasurementLib/Current Measurement  PhasorSimulation=off  OutputType=Complex  PSBequivalent=0
  Diode : spsDiodeLib/Diode  Ron=0.001  Lon=0  Vf=0.8  IC=0  UseSnubber=0  Rs=500  Cs=250e-9  Measurements=on
  IGBT/Diode : spsIGBTDiodeLib/IGBT//Diode  Ron=1e-3  Rs=1e5  Cs=inf  Measurements=on
  Series RLC Branch1 : spsSeriesRLCBranchLib/Series RLC Branch  LConnTagsString=__new0  RConnTagsString=__new0  BranchType=C  Resistance=1e-4  Inductance=200e-6  SetiL0=off  InitialCurrent=0  Capacitance=CoutModulesp  Setx0=off  InitialVoltage=1200  Measurements=None
  Voltage Measurement5 : spsVoltageMeasurementLib/Voltage Measurement  PhasorSimulation=off  OutputType=Complex  PSBequivalent=0
  In+ : PMIOPort  Side=Left
  In- : PMIOPort  Port=2  Side=Left
  Out+ : PMIOPort  Port=3  Side=Right
  Out- : PMIOPort  Port=4  Side=Right
  tag scope: Iinc=global, Voutc=global
  wires:
  [G1c] -> IGBT/Diode/1
  Current Measurement/1 -> [Iinc]
  Voltage Measurement5/1 -> [Voutc]
  connections:
  IGBT/Diode/LConn1 -- Diode/LConn1 -- Current Measurement/RConn1
  Voltage Measurement5/LConn1 -- Out+/RConn1 -- Series RLC Branch1/LConn1 -- Diode/RConn1
  Current Measurement/LConn1 -- In+/RConn1
  Voltage Measurement5/LConn2 -- Out-/RConn1 -- Series RLC Branch1/RConn1 -- In-/RConn1 -- IGBT/Diode/RConn1

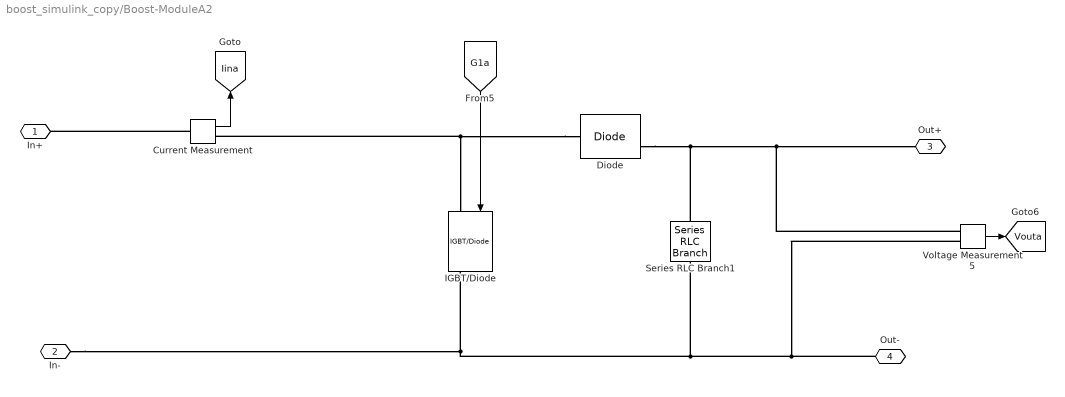
== system boost_simulink_copy/Boost-ModuleA2 ==
  Current Measurement : spsCurrentMeasurementLib/Current Measurement  PhasorSimulation=off  OutputType=Complex  PSBequivalent=0
  Diode : spsDiodeLib/Diode  Ron=0.001  Lon=0  Vf=0.8  IC=0  UseSnubber=0  Rs=500  Cs=250e-9  Measurements=on
  IGBT/Diode : spsIGBTDiodeLib/IGBT//Diode  Ron=1e-3  Rs=1e5  Cs=inf  Measurements=on
  Series RLC Branch1 : spsSeriesRLCBranchLib/Series RLC Branch  LConnTagsString=__new0  RConnTagsString=__new0  BranchType=C  Resistance=1e-4  Inductance=200e-6  SetiL0=off  InitialCurrent=0  Capacitance=CoutModulesp  Setx0=off  InitialVoltage=1200  Measurements=None
  Voltage Measurement5 : spsVoltageMeasurementLib/Voltage Measurement  PhasorSimulation=off  OutputType=Complex  PSBequivalent=0
  In+ : PMIOPort  Side=Left
  In- : PMIOPort  Port=2  Side=Left
  Out+ : PMIOPort  Port=3  Side=Right
  Out- : PMIOPort  Port=4  Side=Right
  tag scope: Iina=global, Vouta=global
  wires:
  [G1a] -> IGBT/Diode/1
  Current Measurement/1 -> [Iina]
  Voltage Measurement5/1 -> [Vouta]
  connections:
  Diode/LConn1 -- IGBT/Diode/LConn1 -- Current Measurement/RConn1
  Series RLC Branch1/LConn1 -- Diode/RConn1 -- Voltage Measurement5/LConn1 -- Out+/RConn1
  Current Measurement/LConn1 -- In+/RConn1
  Out-/RConn1 -- Voltage Measurement5/LConn2 -- In-/RConn1 -- IGBT/Diode/RConn1 -- Series RLC Branch1/RConn1

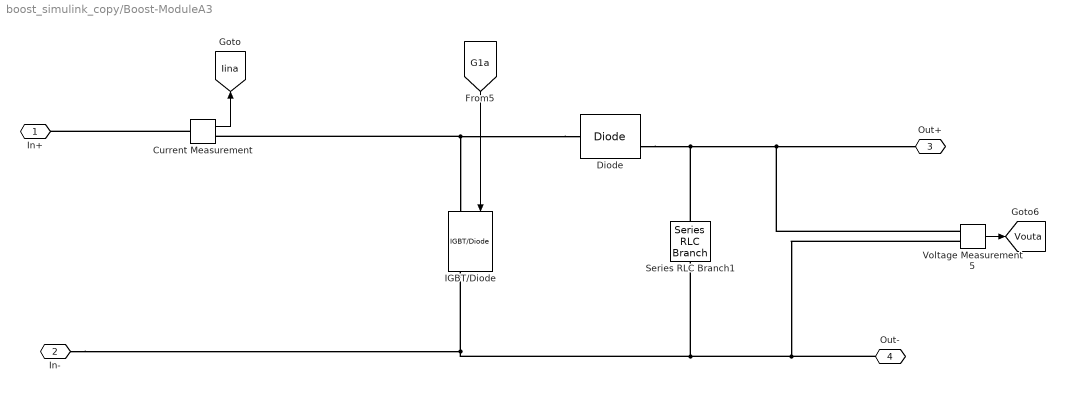
== system boost_simulink_copy/Boost-ModuleA3 ==
  Current Measurement : spsCurrentMeasurementLib/Current Measurement  PhasorSimulation=off  OutputType=Complex  PSBequivalent=0
  Diode : spsDiodeLib/Diode  Ron=0.001  Lon=0  Vf=0.8  IC=0  UseSnubber=0  Rs=500  Cs=250e-9  Measurements=on
  IGBT/Diode : spsIGBTDiodeLib/IGBT//Diode  Ron=1e-3  Rs=1e5  Cs=inf  Measurements=on
  Series RLC Branch1 : spsSeriesRLCBranchLib/Series RLC Branch  LConnTagsString=__new0  RConnTagsString=__new0  BranchType=C  Resistance=1e-4  Inductance=200e-6  SetiL0=off  InitialCurrent=0  Capacitance=CoutModulesp  Setx0=off  InitialVoltage=1200  Measurements=None
  Voltage Measurement5 : spsVoltageMeasurementLib/Voltage Measurement  PhasorSimulation=off  OutputType=Complex  PSBequivalent=0
  In+ : PMIOPort  Side=Left
  In- : PMIOPort  Port=2  Side=Left
  Out+ : PMIOPort  Port=3  Side=Right
  Out- : PMIOPort  Port=4  Side=Right
  tag scope: Iina=global, Vouta=global
  wires:
  [G1a] -> IGBT/Diode/1
  Current Measurement/1 -> [Iina]
  Voltage Measurement5/1 -> [Vouta]
  connections:
  Diode/LConn1 -- IGBT/Diode/LConn1 -- Current Measurement/RConn1
  Series RLC Branch1/LConn1 -- Diode/RConn1 -- Voltage Measurement5/LConn1 -- Out+/RConn1
  Current Measurement/LConn1 -- In+/RConn1
  Out-/RConn1 -- Voltage Measurement5/LConn2 -- In-/RConn1 -- IGBT/Diode/RConn1 -- Series RLC Branch1/RConn1

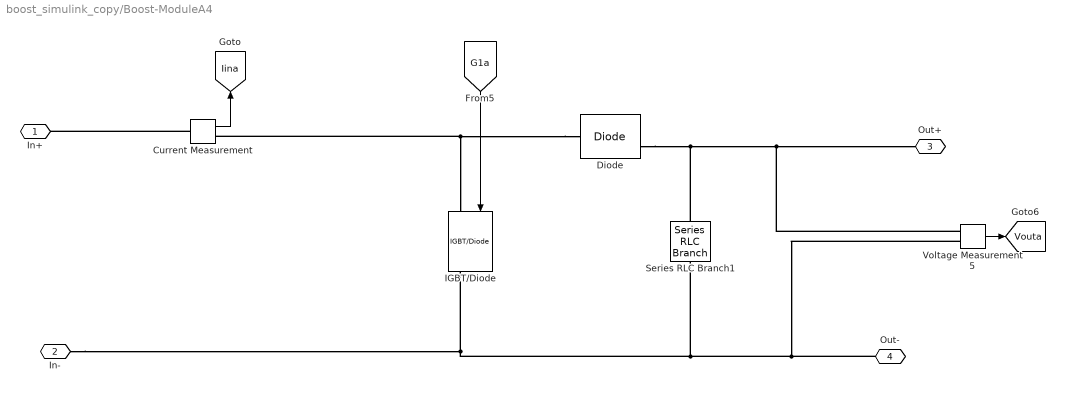
== system boost_simulink_copy/Boost-ModuleA4 ==
  Current Measurement : spsCurrentMeasurementLib/Current Measurement  PhasorSimulation=off  OutputType=Complex  PSBequivalent=0
  Diode : spsDiodeLib/Diode  Ron=0.001  Lon=0  Vf=0.8  IC=0  UseSnubber=0  Rs=500  Cs=250e-9  Measurements=on
  IGBT/Diode : spsIGBTDiodeLib/IGBT//Diode  Ron=1e-3  Rs=1e5  Cs=inf  Measurements=on
  Series RLC Branch1 : spsSeriesRLCBranchLib/Series RLC Branch  LConnTagsString=__new0  RConnTagsString=__new0  BranchType=C  Resistance=1e-4  Inductance=200e-6  SetiL0=off  InitialCurrent=0  Capacitance=CoutModulesp  Setx0=off  InitialVoltage=1200  Measurements=None
  Voltage Measurement5 : spsVoltageMeasurementLib/Voltage Measurement  PhasorSimulation=off  OutputType=Complex  PSBequivalent=0
  In+ : PMIOPort  Side=Left
  In- : PMIOPort  Port=2  Side=Left
  Out+ : PMIOPort  Port=3  Side=Right
  Out- : PMIOPort  Port=4  Side=Right
  tag scope: Iina=global, Vouta=global
  wires:
  [G1a] -> IGBT/Diode/1
  Current Measurement/1 -> [Iina]
  Voltage Measurement5/1 -> [Vouta]
  connections:
  Diode/LConn1 -- IGBT/Diode/LConn1 -- Current Measurement/RConn1
  Series RLC Branch1/LConn1 -- Diode/RConn1 -- Voltage Measurement5/LConn1 -- Out+/RConn1
  Current Measurement/LConn1 -- In+/RConn1
  Out-/RConn1 -- Voltage Measurement5/LConn2 -- In-/RConn1 -- IGBT/Diode/RConn1 -- Series RLC Branch1/RConn1

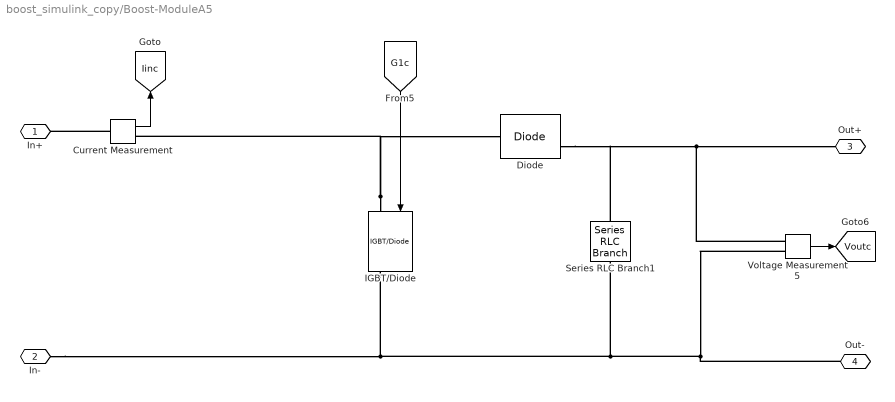
== system boost_simulink_copy/Boost-ModuleA5 ==
  Current Measurement : spsCurrentMeasurementLib/Current Measurement  PhasorSimulation=off  OutputType=Complex  PSBequivalent=0
  Diode : spsDiodeLib/Diode  Ron=0.001  Lon=0  Vf=0.8  IC=0  UseSnubber=0  Rs=500  Cs=250e-9  Measurements=on
  IGBT/Diode : spsIGBTDiodeLib/IGBT//Diode  Ron=1e-3  Rs=1e5  Cs=inf  Measurements=on
  Series RLC Branch1 : spsSeriesRLCBranchLib/Series RLC Branch  LConnTagsString=__new0  RConnTagsString=__new0  BranchType=C  Resistance=1e-4  Inductance=200e-6  SetiL0=off  InitialCurrent=0  Capacitance=CoutModulesp  Setx0=off  InitialVoltage=1200  Measurements=None
  Voltage Measurement5 : spsVoltageMeasurementLib/Voltage Measurement  PhasorSimulation=off  OutputType=Complex  PSBequivalent=0
  In+ : PMIOPort  Side=Left
  In- : PMIOPort  Port=2  Side=Left
  Out+ : PMIOPort  Port=3  Side=Right
  Out- : PMIOPort  Port=4  Side=Right
  tag scope: Iinc=global, Voutc=global
  wires:
  [G1c] -> IGBT/Diode/1
  Current Measurement/1 -> [Iinc]
  Voltage Measurement5/1 -> [Voutc]
  connections:
  IGBT/Diode/LConn1 -- Diode/LConn1 -- Current Measurement/RConn1
  Voltage Measurement5/LConn1 -- Out+/RConn1 -- Series RLC Branch1/LConn1 -- Diode/RConn1
  Current Measurement/LConn1 -- In+/RConn1
  Voltage Measurement5/LConn2 -- Out-/RConn1 -- Series RLC Branch1/RConn1 -- In-/RConn1 -- IGBT/Diode/RConn1

== system boost_simulink_copy/Boost-ModuleB ==
  Current Measurement : spsCurrentMeasurementLib/Current Measurement  PhasorSimulation=off  OutputType=Complex  PSBequivalent=0
  Diode : spsDiodeLib/Diode  Ron=0.001  Lon=0  Vf=0.8  IC=0  UseSnubber=0  Rs=500  Cs=250e-9  Measurements=on
  IGBT/Diode : spsIGBTDiodeLib/IGBT//Diode  Ron=1e-3  Rs=1e5  Cs=inf  Measurements=on
  Series RLC Branch1 : spsSeriesRLCBranchLib/Series RLC Branch  LConnTagsString=__new0  RConnTagsString=__new0  BranchType=C  Resistance=1e-4  Inductance=200e-6  SetiL0=off  InitialCurrent=0  Capacitance=CoutModulesp  Setx0=off  InitialVoltage=1200  Measurements=None
  Voltage Measurement6 : spsVoltageMeasurementLib/Voltage Measurement  PhasorSimulation=off  OutputType=Complex  PSBequivalent=0
  In+ : PMIOPort  Side=Left
  In- : PMIOPort  Port=2  Side=Left
  Out+ : PMIOPort  Port=3  Side=Right
  Out- : PMIOPort  Port=4  Side=Right
  tag scope: Iinb=global, Voutb=global
  wires:
  Current Measurement/1 -> [Iinb]
  [G1b] -> IGBT/Diode/1
  Voltage Measurement6/1 -> [Voutb]
  connections:
  Out+/RConn1 -- Voltage Measurement6/LConn1 -- Series RLC Branch1/LConn1 -- Current Measurement/RConn1 -- IGBT/Diode/LConn1
  Out-/RConn1 -- Voltage Measurement6/LConn2 -- Diode/LConn1 -- Series RLC Branch1/RConn1
  Current Measurement/LConn1 -- In+/RConn1
  In-/RConn1 -- Diode/RConn1 -- IGBT/Diode/RConn1

== system boost_simulink_copy/Boost-ModuleB1 ==
  Current Measurement : spsCurrentMeasurementLib/Current Measurement  PhasorSimulation=off  OutputType=Complex  PSBequivalent=0
  Diode : spsDiodeLib/Diode  Ron=0.001  Lon=0  Vf=0.8  IC=0  UseSnubber=0  Rs=500  Cs=250e-9  Measurements=on
  IGBT/Diode : spsIGBTDiodeLib/IGBT//Diode  Ron=1e-3  Rs=1e5  Cs=inf  Measurements=on
  Series RLC Branch1 : spsSeriesRLCBranchLib/Series RLC Branch  LConnTagsString=__new0  RConnTagsString=__new0  BranchType=C  Resistance=1e-4  Inductance=200e-6  SetiL0=off  InitialCurrent=0  Capacitance=CoutModulesp  Setx0=off  InitialVoltage=1200  Measurements=None
  Voltage Measurement6 : spsVoltageMeasurementLib/Voltage Measurement  PhasorSimulation=off  OutputType=Complex  PSBequivalent=0
  In+ : PMIOPort  Side=Left
  In- : PMIOPort  Port=2  Side=Left
  Out+ : PMIOPort  Port=3  Side=Right
  Out- : PMIOPort  Port=4  Side=Right
  tag scope: Iind=global, Voutd=global
  wires:
  Current Measurement/1 -> [Iind]
  [G1d] -> IGBT/Diode/1
  Voltage Measurement6/1 -> [Voutd]
  connections:
  Current Measurement/RConn1 -- IGBT/Diode/LConn1 -- Series RLC Branch1/LConn1 -- Voltage Measurement6/LConn1 -- Out+/RConn1
  Diode/LConn1 -- Series RLC Branch1/RConn1 -- Out-/RConn1 -- Voltage Measurement6/LConn2
  Current Measurement/LConn1 -- In+/RConn1
  In-/RConn1 -- IGBT/Diode/RConn1 -- Diode/RConn1

== system boost_simulink_copy/Boost-ModuleB2 ==
  Current Measurement : spsCurrentMeasurementLib/Current Measurement  PhasorSimulation=off  OutputType=Complex  PSBequivalent=0
  Diode : spsDiodeLib/Diode  Ron=0.001  Lon=0  Vf=0.8  IC=0  UseSnubber=0  Rs=500  Cs=250e-9  Measurements=on
  IGBT/Diode : spsIGBTDiodeLib/IGBT//Diode  Ron=1e-3  Rs=1e5  Cs=inf  Measurements=on
  Series RLC Branch1 : spsSeriesRLCBranchLib/Series RLC Branch  LConnTagsString=__new0  RConnTagsString=__new0  BranchType=C  Resistance=1e-4  Inductance=200e-6  SetiL0=off  InitialCurrent=0  Capacitance=CoutModulesp  Setx0=off  InitialVoltage=1200  Measurements=None
  Voltage Measurement6 : spsVoltageMeasurementLib/Voltage Measurement  PhasorSimulation=off  OutputType=Complex  PSBequivalent=0
  In+ : PMIOPort  Side=Left
  In- : PMIOPort  Port=2  Side=Left
  Out+ : PMIOPort  Port=3  Side=Right
  Out- : PMIOPort  Port=4  Side=Right
  tag scope: Iinb=global, Voutb=global
  wires:
  Current Measurement/1 -> [Iinb]
  [G1b] -> IGBT/Diode/1
  Voltage Measurement6/1 -> [Voutb]
  connections:
  Out+/RConn1 -- Voltage Measurement6/LConn1 -- Series RLC Branch1/LConn1 -- Current Measurement/RConn1 -- IGBT/Diode/LConn1
  Out-/RConn1 -- Voltage Measurement6/LConn2 -- Diode/LConn1 -- Series RLC Branch1/RConn1
  Current Measurement/LConn1 -- In+/RConn1
  In-/RConn1 -- Diode/RConn1 -- IGBT/Diode/RConn1

== system boost_simulink_copy/PWM Block  ==
  AND : Logic  IconShape=distinctive  AllPortsSameDT=off  OutDataTypeStr=boolean
  AND1 : Logic  IconShape=distinctive  AllPortsSameDT=off  OutDataTypeStr=boolean
  Compare To Zero : simulink/Logic and Bit Operations/Compare To Zero  relop=>  OutDataTypeStr=boolean
  Compare To Zero3 : simulink/Logic and Bit Operations/Compare To Zero  relop=<  OutDataTypeStr=boolean
  Constant : Constant  Value=2*D-1
  Delay : Delay
  Delay1 : Delay
  Subtract : Sum  Inputs=+-
  Triangle Generator : spsTriangleGeneratorLib/Triangle Generator  Freq=fsw  Phase=ModuleAPhase  Ts=sampleTime
  tag scope: G1a=global, G2a=global
  wires:
  Constant/1 -> Subtract/1
  Triangle Generator/1 -> Subtract/2
  Subtract/1 -> Compare To Zero3/1, Compare To Zero/1
  AND/1 -> [G1a]
  Compare To Zero/1 -> Delay/1, AND/2
  Delay/1 -> AND/1
  Compare To Zero3/1 -> Delay1/1, AND1/1  "ab"
  AND1/1 -> [G2a]
  Delay1/1 -> AND1/2

== system boost_simulink_copy/PWM Block - 1 ==
  AND : Logic  IconShape=distinctive  AllPortsSameDT=off  OutDataTypeStr=boolean
  AND1 : Logic  IconShape=distinctive  AllPortsSameDT=off  OutDataTypeStr=boolean
  Compare To Zero : simulink/Logic and Bit Operations/Compare To Zero  relop=>  OutDataTypeStr=boolean
  Compare To Zero3 : simulink/Logic and Bit Operations/Compare To Zero  relop=<  OutDataTypeStr=boolean
  Constant : Constant  Value=2*D-1
  Delay : Delay
  Delay1 : Delay
  Subtract : Sum  Inputs=+-
  Triangle Generator : spsTriangleGeneratorLib/Triangle Generator  Freq=fsw  Phase=ModuleAPhase  Ts=sampleTime
  tag scope: G1a=global, G2a=global
  wires:
  Constant/1 -> Subtract/1
  Triangle Generator/1 -> Subtract/2
  Subtract/1 -> Compare To Zero3/1, Compare To Zero/1
  AND/1 -> [G1a]
  Compare To Zero/1 -> Delay/1, AND/2
  Delay/1 -> AND/1
  Compare To Zero3/1 -> Delay1/1, AND1/1  "ab"
  AND1/1 -> [G2a]
  Delay1/1 -> AND1/2

== system boost_simulink_copy/PWM Block - 2 ==
  AND : Logic  IconShape=distinctive  AllPortsSameDT=off  OutDataTypeStr=boolean
  AND1 : Logic  IconShape=distinctive  AllPortsSameDT=off  OutDataTypeStr=boolean
  Compare To Zero : simulink/Logic and Bit Operations/Compare To Zero  relop=>  OutDataTypeStr=boolean
  Compare To Zero3 : simulink/Logic and Bit Operations/Compare To Zero  relop=<  OutDataTypeStr=boolean
  Constant : Constant  Value=2*D-1
  Delay : Delay
  Delay1 : Delay
  Subtract : Sum  Inputs=+-
  Triangle Generator : spsTriangleGeneratorLib/Triangle Generator  Freq=fsw  Phase=ModuleBPhase  Ts=sampleTime
  tag scope: G1b=global, G2b=global
  wires:
  Constant/1 -> Subtract/1
  Triangle Generator/1 -> Subtract/2
  Subtract/1 -> Compare To Zero3/1, Compare To Zero/1
  AND/1 -> [G1b]
  Compare To Zero/1 -> Delay/1, AND/2
  Delay/1 -> AND/1
  Compare To Zero3/1 -> Delay1/1, AND1/1  "ab"
  AND1/1 -> [G2b]
  Delay1/1 -> AND1/2

== system boost_simulink_copy/PWM Block2 ==
  AND : Logic  IconShape=distinctive  AllPortsSameDT=off  OutDataTypeStr=boolean
  AND1 : Logic  IconShape=distinctive  AllPortsSameDT=off  OutDataTypeStr=boolean
  Compare To Zero : simulink/Logic and Bit Operations/Compare To Zero  relop=>  OutDataTypeStr=boolean
  Compare To Zero3 : simulink/Logic and Bit Operations/Compare To Zero  relop=<  OutDataTypeStr=boolean
  Constant : Constant  Value=2*D-1
  Delay : Delay
  Delay1 : Delay
  Subtract : Sum  Inputs=+-
  Triangle Generator : spsTriangleGeneratorLib/Triangle Generator  Freq=fsw  Phase=ModuleCPhase  Ts=sampleTime
  tag scope: G1c=global, G2c=global
  wires:
  Constant/1 -> Subtract/1
  Triangle Generator/1 -> Subtract/2
  Subtract/1 -> Compare To Zero3/1, Compare To Zero/1
  AND/1 -> [G1c]
  Compare To Zero/1 -> Delay/1, AND/2
  Delay/1 -> AND/1
  Compare To Zero3/1 -> Delay1/1, AND1/1  "ab"
  AND1/1 -> [G2c]
  Delay1/1 -> AND1/2

== system boost_simulink_copy/PWM Block3 ==
  AND : Logic  IconShape=distinctive  AllPortsSameDT=off  OutDataTypeStr=boolean
  AND1 : Logic  IconShape=distinctive  AllPortsSameDT=off  OutDataTypeStr=boolean
  Compare To Zero : simulink/Logic and Bit Operations/Compare To Zero  relop=>  OutDataTypeStr=boolean
  Compare To Zero3 : simulink/Logic and Bit Operations/Compare To Zero  relop=<  OutDataTypeStr=boolean
  Constant : Constant  Value=2*D-1
  Delay : Delay
  Delay1 : Delay
  Subtract : Sum  Inputs=+-
  Triangle Generator : spsTriangleGeneratorLib/Triangle Generator  Freq=fsw  Phase=ModuleDPhase  Ts=sampleTime
  tag scope: G1d=global, G2d=global
  wires:
  Constant/1 -> Subtract/1
  Triangle Generator/1 -> Subtract/2
  Subtract/1 -> Compare To Zero3/1, Compare To Zero/1
  AND/1 -> [G1d]
  Compare To Zero/1 -> Delay/1, AND/2
  Delay/1 -> AND/1
  Compare To Zero3/1 -> Delay1/1, AND1/1  "ab"
  AND1/1 -> [G2d]
  Delay1/1 -> AND1/2
